simulink model "third_order"  (R2021b)
settings: Solver=VariableStepAuto  StartTime=0.0  StopTime=20  RelTol=1e-3
undefined symbols (not defined in the file): Amax, Amin, Ts, U, Vmax, Vmin
settings Model: Creator=11035  LastModifiedBy=11035

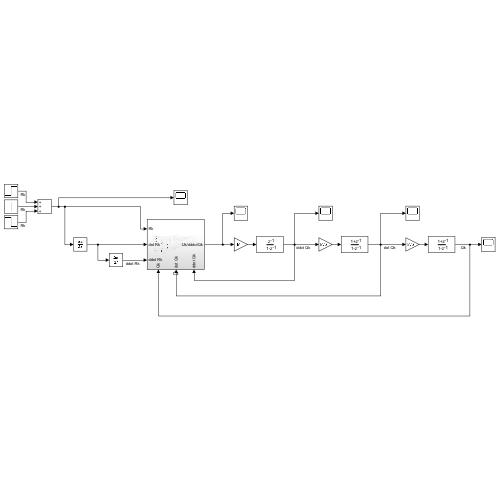
[thumbnail: Simulink's stored preview of the top-level diagram]
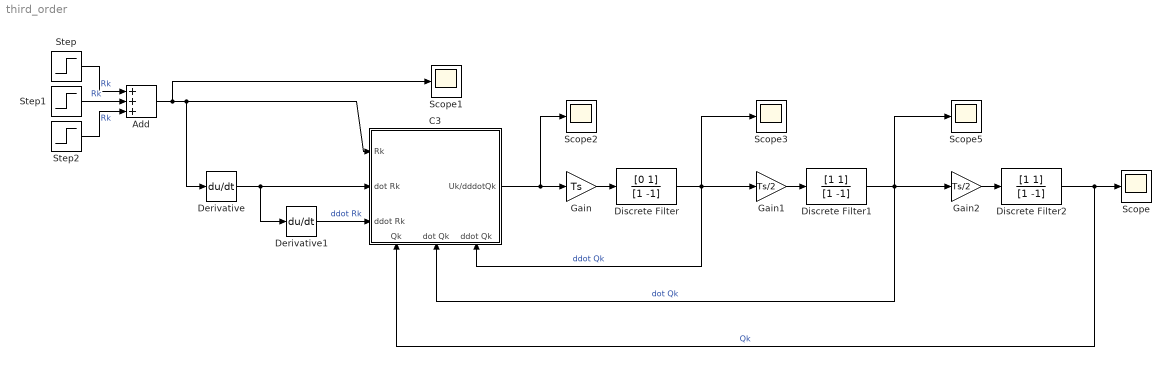
== system third_order ==
  Add : Sum  Inputs=+++
  C3 : Subsystem
      settings: PortSchema="{\"entries\":[{\"content\":{\"sides\":[{\"content\":{\"connectorIds\":[\"In1\",\"In2\",\"In3\"]},\"type\":\"ConnectorPlacement.EquallySpacedRectSide\",\"uuid\":\"716dbc1c-49b2-4cb8-9978-582acac14571\"},{\"content\":{\"connectorIds\":[\"Out1\"],\"side\":\"RIGHT\"},\"type\":\"ConnectorPlacement.EquallySpacedRectSide\",\"uuid\":\"02ab29e9-5fcc-4cd5-9c74-177b5082cb9c\"},{\"content\":{\"connectorIds\":[],\"side\":\"TOP\"},\"type\":\"ConnectorPlacement.EquallySpacedRectSide\",\"uuid\":\"01e65ab7-ae67-4bc4-815c-31b93fbda65a\"},{\"content\":{\"connectorIds\":[\"In4\",\"In5\",\"In6\"],\"side\":\"BOTTOM\"},\"type\":\"ConnectorPlacement.EquallySpacedRectSide\",\"uuid\":\"7a24d1a6-7a93-4ed1-ab59-9b35f53416c1\"}]},\"type\":\"ConnectorPlacement.EquallySpacedConnector\",\"uuid\":\"504bdbd8-79dc-4418-b775-c54dc6ccf1a1\"}],\"packageUris\":[\"http://schema.mathworks.com/mf0/Connector/R2020b\"],\"version\":\"1.0\"}"
  Derivative : Derivative
  Derivative1 : Derivative
  Discrete Filter : DiscreteFilter  Numerator=[0 1]  Denominator=[1 -1]
  Discrete Filter1 : DiscreteFilter  Numerator=[1 1]  Denominator=[1 -1]
  Discrete Filter2 : DiscreteFilter  Numerator=[1 1]  Denominator=[1 -1]
  Gain : Gain  Gain=Ts
  Gain1 : Gain  Gain=Ts/2
  Gain2 : Gain  Gain=Ts/2
  Scope{,1..3,5} (5 alike) : Scope
  Step : Step  After=4  SampleTime=0.001
  Step1 : Step  Time=7  After=6  SampleTime=0.001
  Step2 : Step  Time=13  After=-12  SampleTime=0.001
  wires:
  Gain1/1 -> Discrete Filter1/1
  Gain/1 -> Discrete Filter/1
  Discrete Filter1/1 -> C3/5(dot Qk), Gain2/1, Scope5/1  "dot Qk"
  Discrete Filter/1 -> C3/6(ddot Qk), Scope3/1, Gain1/1  "ddot Qk"
  Gain2/1 -> Discrete Filter2/1
  Discrete Filter2/1 -> Scope/1, C3/4(Qk)  "Qk"
  C3/1(Uk/dddotQk) -> Scope2/1, Gain/1
  Step1/1 -> Add/2  "Rk"
  Step/1 -> Add/1  "Rk"
  Step2/1 -> Add/3  "Rk"
  Add/1 -> Scope1/1, Derivative/1, C3/1(Rk)
  Derivative/1 -> C3/2(dot Rk), Derivative1/1
  Derivative1/1 -> C3/3(ddot Rk)  "ddot Rk"

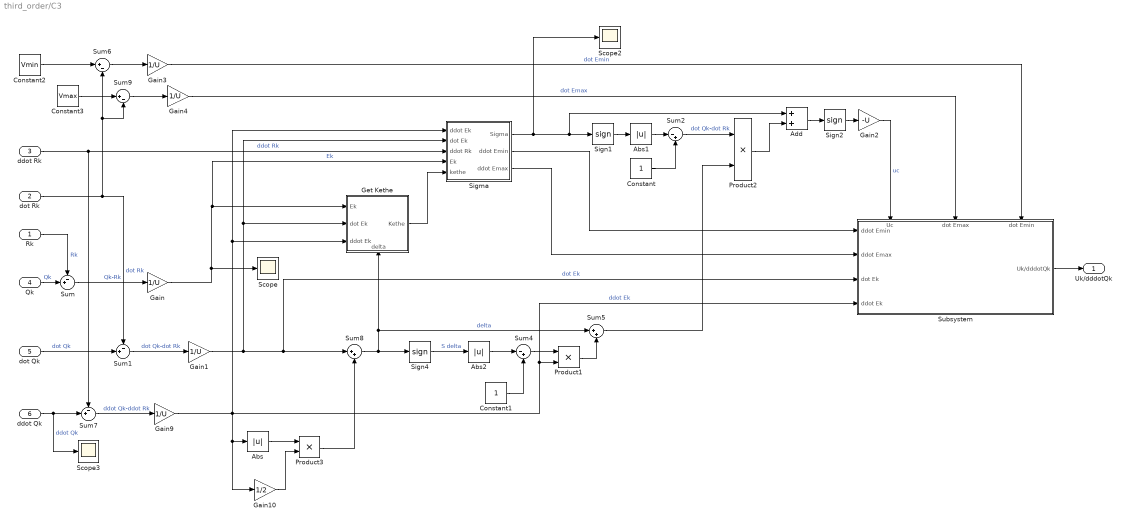
== system third_order/C3 ==
  Rk : Inport
  dot Rk : Inport  Port=2
  ddot Rk : Inport  Port=3
  Qk : Inport  Port=4
  dot Qk : Inport  Port=5
  ddot Qk : Inport  Port=6
  Abs : Abs
  Abs1 : Abs
  Abs2 : Abs
  Add : Sum
  Constant : Constant
  Constant1 : Constant
  Constant2 : Constant  Value=Vmin
  Constant3 : Constant  Value=Vmax
  Gain{,1,3..4,9} (5 alike) : Gain  Gain=1/U
  Gain10 : Gain  Gain=1/2
  Gain2 : Gain  Gain=-U
  Get Kethe : Subsystem
      settings: PortSchema="{\"entries\":[{\"content\":{\"sides\":[{\"content\":{\"connectorIds\":[\"In1\",\"In2\",\"In3\"]},\"type\":\"ConnectorPlacement.EquallySpacedRectSide\",\"uuid\":\"9252580f-5e9d-4265-be0b-e6bb3d304b20\"},{\"content\":{\"connectorIds\":[\"Out1\"],\"side\":\"RIGHT\"},\"type\":\"ConnectorPlacement.EquallySpacedRectSide\",\"uuid\":\"31fc0c8b-d7d5-4d3b-a162-fba5885efc54\"},{\"content\":{\"connectorIds\":[],\"side\":\"TOP\"},\"type\":\"ConnectorPlacement.EquallySpacedRectSide\",\"uuid\":\"1870fd8d-4272-45e5-86fe-422e41d939fb\"},{\"content\":{\"connectorIds\":[\"In4\"],\"side\":\"BOTTOM\"},\"type\":\"ConnectorPlacement.EquallySpacedRectSide\",\"uuid\":\"f1cc4331-f119-4651-8dc3-66dcf886f7f7\"}]},\"type\":\"ConnectorPlacement.EquallySpacedConnector\",\"uuid\":\"c093638c-209e-48b2-8550-858719cb62f2\"}],\"packageUris\":[\"http://schema.mathworks.com/mf0/Connector/R2020b\"],\"version\":\"1.0\"}"
  Product1 : Product
  Product2 : Product
  Product3 : Product
  Scope : Scope
  Scope2 : Scope
  Scope3 : Scope
  Sigma : Subsystem
  Sign1 : Signum
  Sign2 : Signum
  Sign4 : Signum
  Subsystem : Subsystem
      settings: PortSchema="{\"entries\":[{\"content\":{\"sides\":[{\"content\":{\"connectorIds\":[\"In1\",\"In2\",\"In3\",\"In4\"]},\"type\":\"ConnectorPlacement.EquallySpacedRectSide\",\"uuid\":\"36f01cd8-9b20-4b96-874e-21a8302aaf05\"},{\"content\":{\"connectorIds\":[\"Out1\"],\"side\":\"RIGHT\"},\"type\":\"ConnectorPlacement.EquallySpacedRectSide\",\"uuid\":\"aff3e783-8ccd-4767-9c32-464e65717a87\"},{\"content\":{\"connectorIds\":[\"In5\",\"In6\",\"In7\"],\"side\":\"TOP\"},\"type\":\"ConnectorPlacement.EquallySpacedRectSide\",\"uuid\":\"c94c5949-abb6-4ff8-bb3f-d90959b8a55f\"}]},\"type\":\"ConnectorPlacement.EquallySpacedConnector\",\"uuid\":\"91cab301-bc0d-448e-a06d-cf998fceab8f\"}],\"packageUris\":[\"http://schema.mathworks.com/mf0/Connector/R2020b\"],\"version\":\"1.0\"}"
  Sum : Sum  Inputs=-+|
  Sum1 : Sum  Inputs=-+|
  Sum2 : Sum  Inputs=|-+
  Sum4 : Sum  Inputs=|-+
  Sum5 : Sum  Inputs=|++
  Sum6 : Sum  Inputs=|+-
  Sum7 : Sum  Inputs=-+|
  Sum8 : Sum  Inputs=|++
  Sum9 : Sum  Inputs=|+-
  Uk/dddotQk : Outport
  wires:
  Rk/1 -> Sum/1  "Rk"
  Qk/1 -> Sum/2  "Qk"
  Sum/1 -> Gain/1  "Qk-Rk"
  dot Qk/1 -> Sum1/2  "dot Qk"
  Sum1/1 -> Gain1/1  "dot Qk-dot Rk"
  dot Rk/1 -> Sum9/2, Sum6/2, Sum1/1  "dot Rk"
  ddot Qk/1 -> Scope3/1, Sum7/2  "ddot Qk"
  Sum7/1 -> Gain9/1  "ddot Qk-ddot Rk"
  Abs/1 -> Product3/1
  Gain10/1 -> Product3/2
  Product3/1 -> Sum8/2
  Sum8/1 -> Sign4/1, Sum5/1, Get Kethe/4(delta)  "delta"
  Sign4/1 -> Abs2/1  "S delta"
  Gain1/1 -> Sigma/2(dot Ek), Get Kethe/2(dot Ek), Sum8/1, Subsystem/3(dot Ek)  "dot Ek"
  Gain9/1 -> Gain10/1, Abs/1, Product1/2, Subsystem/4(ddot Ek), Get Kethe/3(ddot Ek), Sigma/1(ddot Ek)  "ddot Ek"
  ddot Rk/1 -> Sum7/1, Sigma/3(ddot Rk)  "ddot Rk"
  Gain/1 -> Scope/1, Sigma/4(Ek), Get Kethe/1(Ek)  "Ek"
  Sigma/1(Sigma) -> Scope2/1, Add/1, Sign1/1
  Sign1/1 -> Abs1/1
  Abs1/1 -> Sum2/1
  Constant/1 -> Sum2/2
  Constant1/1 -> Sum4/2
  Abs2/1 -> Sum4/1
  Sum4/1 -> Product1/1
  Product1/1 -> Sum5/2
  Sigma/2(ddot Emin) -> Subsystem/1(ddot Emin)
  Sigma/3(ddot Emax) -> Subsystem/2(ddot Emax)
  Subsystem/1(Uk/dddotQk) -> Uk/dddotQk/1
  Constant2/1 -> Sum6/1
  Sum6/1 -> Gain3/1
  Gain3/1 -> Subsystem/7(dot Emin)  "dot Emin"
  Constant3/1 -> Sum9/1
  Sum9/1 -> Gain4/1
  Gain4/1 -> Subsystem/6(dot Emax)  "dot Emax"
  Sum2/1 -> Product2/1  "dot Qk-dot Rk"
  Sum5/1 -> Product2/2
  Product2/1 -> Add/2
  Add/1 -> Sign2/1
  Gain2/1 -> Subsystem/5("Uc ")  "uc"
  Get Kethe/1(Kethe) -> Sigma/5(kethe)
  Sign2/1 -> Gain2/1

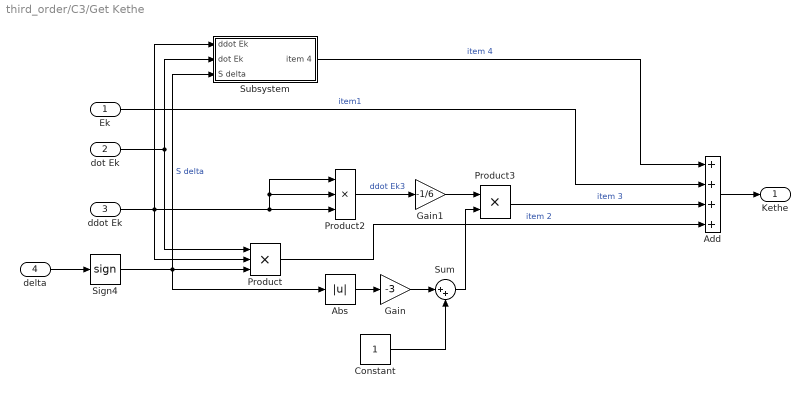
== system third_order/C3/Get Kethe ==
  Ek : Inport
  dot Ek : Inport  Port=2
  ddot Ek : Inport  Port=3
  delta : Inport  Port=4
  Abs : Abs
  Add : Sum  Inputs=++++
  Constant : Constant
  Gain : Gain  Gain=-3
  Gain1 : Gain  Gain=-1/6
  Product : Product  Inputs=3
  Product2 : Product  Inputs=3
  Product3 : Product
  Sign4 : Signum
  Subsystem : Subsystem
  Sum : Sum  Inputs=|++
  Kethe : Outport
  wires:
  delta/1 -> Sign4/1
  dot Ek/1 -> Subsystem/2(dot Ek), Product/1
  ddot Ek/1 -> Product2/2, Product2/1, Product2/3, Subsystem/1(ddot Ek), Product/2
  Product2/1 -> Gain1/1  "ddot Ek3"
  Product/1 -> Add/4  "item 2"
  Sign4/1 -> Subsystem/3(S delta), Product/3, Abs/1  "S delta"
  Abs/1 -> Gain/1
  Gain/1 -> Sum/1
  Constant/1 -> Sum/2
  Gain1/1 -> Product3/1
  Sum/1 -> Product3/2
  Product3/1 -> Add/3  "item 3"
  Subsystem/1(item 4) -> Add/1  "item 4"
  Ek/1 -> Add/2  "item1"
  Add/1 -> Kethe/1

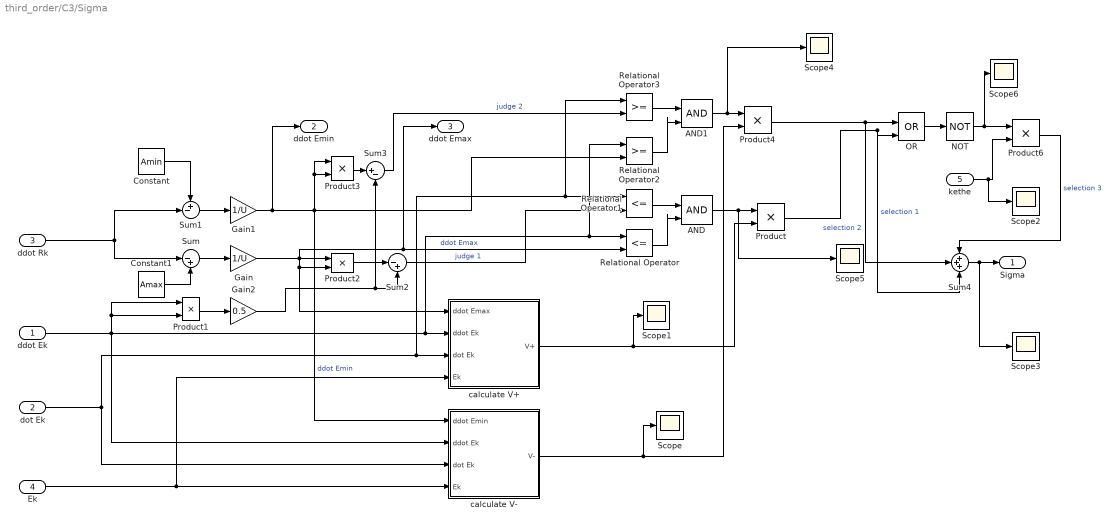
== system third_order/C3/Sigma ==
  ddot Ek : Inport
  dot Ek : Inport  Port=2
  ddot Rk : Inport  Port=3
  Ek : Inport  Port=4
  kethe : Inport  Port=5
  AND : Logic  IconShape=distinctive  AllPortsSameDT=off  OutDataTypeStr=boolean
  AND1 : Logic  IconShape=distinctive  AllPortsSameDT=off  OutDataTypeStr=boolean
  Constant : Constant  Value=Amin
  Constant1 : Constant  Value=Amax
  Gain : Gain  Gain=1/U
  Gain1 : Gain  Gain=1/U
  Gain2 : Gain  Gain=0.5
  NOT : Logic  Operator=NOT  IconShape=distinctive  AllPortsSameDT=off  OutDataTypeStr=boolean
  OR : Logic  Operator=OR  IconShape=distinctive  AllPortsSameDT=off  OutDataTypeStr=boolean
  Product{,1..4,6} (6 alike) : Product
  Relational Operator : RelationalOperator  Operator=<=  OutDataTypeStr=boolean  RndMeth=Simplest
  Relational Operator1 : RelationalOperator  Operator=<=  OutDataTypeStr=boolean  RndMeth=Simplest
  Relational Operator2 : RelationalOperator  OutDataTypeStr=boolean  RndMeth=Simplest
  Relational Operator3 : RelationalOperator  OutDataTypeStr=boolean  RndMeth=Simplest
  Scope{,1..6} (7 alike) : Scope
  Sum : Sum  Inputs=|-+
  Sum1 : Sum  Inputs=+-|
  Sum2 : Sum  Inputs=|-+
  Sum3 : Sum  Inputs=|+-
  Sum4 : Sum  Inputs=+++
  calculate V+ : Subsystem
  calculate V- : Subsystem
  Sigma : Outport
  ddot Emin : Outport  Port=2
  ddot Emax : Outport  Port=3
  wires:
  Sum1/1 -> Gain1/1
  Constant/1 -> Sum1/1
  Sum/1 -> Gain/1
  ddot Rk/1 -> Sum/1, Sum1/2
  Constant1/1 -> Sum/2
  dot Ek/1 -> calculate V-/3(dot Ek), Relational Operator3/1, Relational Operator1/1, calculate V+/3(dot Ek)
  Ek/1 -> calculate V-/4(Ek), calculate V+/4(Ek)
  Gain1/1 -> Relational Operator2/2, Product3/2, Product3/1, calculate V-/1(ddot Emin), ddot Emin/1  "ddot Emin"
  Gain/1 -> Product2/1, calculate V+/1(ddot Emax), Product2/2, ddot Emax/1, Relational Operator/2  "ddot Emax"
  Product1/1 -> Gain2/1
  Product2/1 -> Sum2/1
  Gain2/1 -> Sum3/2, Sum2/2
  calculate V+/1(V+) -> Scope1/1, Product/2
  Sum2/1 -> Relational Operator1/2  "judge 1"
  Product3/1 -> Sum3/1
  Sum3/1 -> Relational Operator3/2  "judge 2"
  calculate V-/1(V-) -> Scope/1, Product4/2
  ddot Ek/1 -> Product1/1, Product1/2, Relational Operator2/1, Relational Operator/1, calculate V+/2(ddot Ek), calculate V-/2(ddot Ek)
  Relational Operator1/1 -> AND/1
  Relational Operator/1 -> AND/2
  AND/1 -> Scope5/1, Product/1
  Product/1 -> Sum4/3, OR/2  "selection 1"
  Relational Operator3/1 -> AND1/1
  Relational Operator2/1 -> AND1/2
  AND1/1 -> Scope4/1, Product4/1
  OR/1 -> NOT/1
  NOT/1 -> Scope6/1, Product6/1
  kethe/1 -> Scope2/1, Product6/2
  Product6/1 -> Sum4/1  "selection 3"
  Product4/1 -> Sum4/2, OR/1  "selection 2"
  Sum4/1 -> Scope3/1, Sigma/1

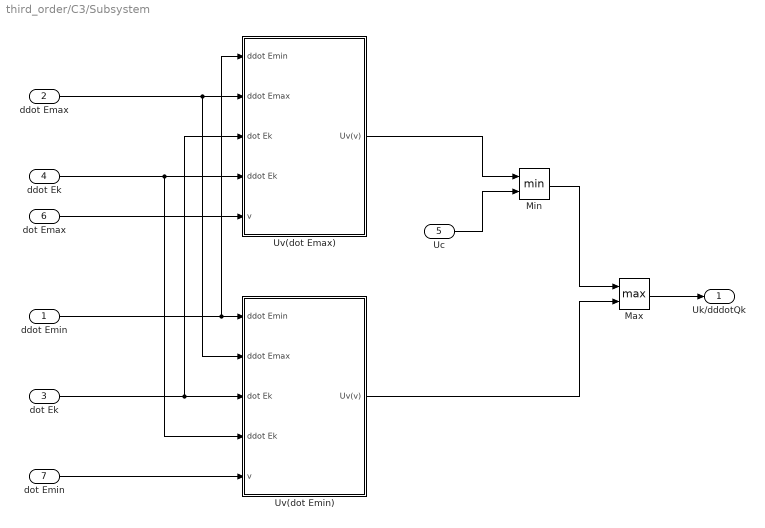
== system third_order/C3/Subsystem ==
  ddot Emin : Inport
  ddot Emax : Inport  Port=2
  dot Ek : Inport  Port=3
  ddot Ek : Inport  Port=4
  "Uc " : Inport  Port=5
  dot Emax : Inport  Port=6
  dot Emin : Inport  Port=7
  Max : MinMax  Function=max  Inputs=2
  Min : MinMax  Inputs=2
  Uv(dot Emax) : Subsystem
  Uv(dot Emin) : Subsystem
  Uk/dddotQk : Outport
  wires:
  ddot Emin/1 -> Uv(dot Emax)/1(ddot Emin), Uv(dot Emin)/1(ddot Emin)
  ddot Emax/1 -> Uv(dot Emin)/2(ddot Emax), Uv(dot Emax)/2(ddot Emax)
  dot Ek/1 -> Uv(dot Emin)/3(dot Ek), Uv(dot Emax)/3(dot Ek)
  ddot Ek/1 -> Uv(dot Emin)/4(ddot Ek), Uv(dot Emax)/4(ddot Ek)
  "Uc "/1 -> Min/2
  Uv(dot Emax)/1(Uv(v)) -> Min/1
  Min/1 -> Max/1
  Uv(dot Emin)/1(Uv(v)) -> Max/2
  Max/1 -> Uk/dddotQk/1
  dot Emax/1 -> Uv(dot Emax)/5("v ")
  dot Emin/1 -> Uv(dot Emin)/5("v ")

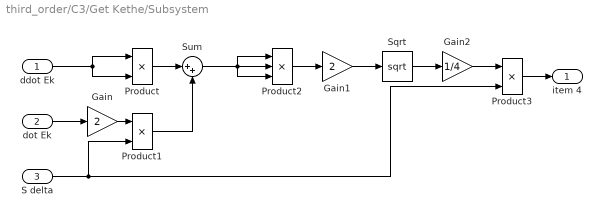
== system third_order/C3/Get Kethe/Subsystem ==
  ddot Ek : Inport
  dot Ek : Inport  Port=2
  S delta : Inport  Port=3
  Gain : Gain  Gain=2
  Gain1 : Gain  Gain=2
  Gain2 : Gain  Gain=1/4
  Product : Product
  Product1 : Product
  Product2 : Product  Inputs=3
  Product3 : Product
  Sqrt : Sqrt  SaturateOnIntegerOverflow=on
  Sum : Sum  Inputs=|++
  item 4 : Outport
  wires:
  ddot Ek/1 -> Product/1, Product/2
  dot Ek/1 -> Gain/1
  Gain/1 -> Product1/1
  S delta/1 -> Product3/2, Product1/2
  Product/1 -> Sum/1
  Product1/1 -> Sum/2
  Sum/1 -> Product2/3, Product2/1, Product2/2
  Product2/1 -> Gain1/1
  Gain1/1 -> Sqrt/1
  Sqrt/1 -> Gain2/1
  Gain2/1 -> Product3/1
  Product3/1 -> item 4/1

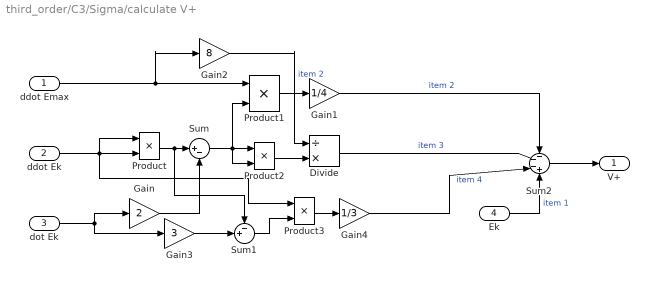
== system third_order/C3/Sigma/calculate V+ ==
  ddot Emax : Inport
  ddot Ek : Inport  Port=2
  dot Ek : Inport  Port=3
  Ek : Inport  Port=4
  Divide : Product  Inputs=/*
  Gain : Gain  Gain=2
  Gain1 : Gain  Gain=1/4
  Gain2 : Gain  Gain=8
  Gain3 : Gain  Gain=3
  Gain4 : Gain  Gain=1/3
  Product{,1..3} (4 alike) : Product
  Sum : Sum  Inputs=|+-
  Sum1 : Sum  Inputs=-+|
  Sum2 : Sum  Inputs=---+
  V+ : Outport
  wires:
  Ek/1 -> Sum2/4  "item 1"
  ddot Ek/1 -> Product3/1, Product/2, Product/1
  Product/1 -> Sum1/1, Sum/1
  Gain/1 -> Sum/2
  ddot Emax/1 -> Gain2/1, Product1/1
  Product1/1 -> Gain1/1
  Gain1/1 -> Sum2/1  "item 2"
  Sum/1 -> Product1/2, Product2/2, Product2/1
  Product2/1 -> Divide/2
  Gain2/1 -> Divide/1  "item 2"
  Divide/1 -> Sum2/2  "item 3"
  dot Ek/1 -> Gain/1, Gain3/1
  Gain3/1 -> Sum1/2
  Sum1/1 -> Product3/2
  Product3/1 -> Gain4/1
  Gain4/1 -> Sum2/3  "item 4"
  Sum2/1 -> V+/1

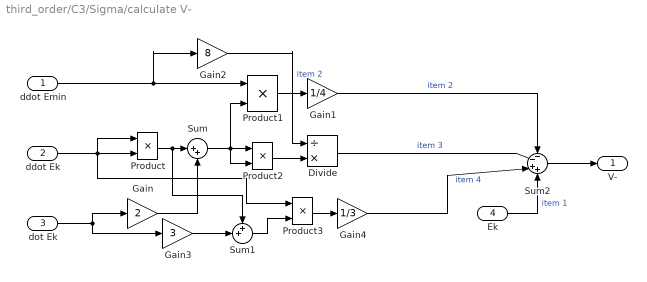
== system third_order/C3/Sigma/calculate V- ==
  ddot Emin : Inport
  ddot Ek : Inport  Port=2
  dot Ek : Inport  Port=3
  Ek : Inport  Port=4
  Divide : Product  Inputs=/*
  Gain : Gain  Gain=2
  Gain1 : Gain  Gain=1/4
  Gain2 : Gain  Gain=8
  Gain3 : Gain  Gain=3
  Gain4 : Gain  Gain=1/3
  Product{,1..3} (4 alike) : Product
  Sum : Sum  Inputs=|++
  Sum1 : Sum  Inputs=++|
  Sum2 : Sum  Inputs=--++
  V- : Outport
  wires:
  Ek/1 -> Sum2/4  "item 1"
  Product/1 -> Sum1/1, Sum/1
  Gain/1 -> Sum/2
  ddot Emin/1 -> Gain2/1, Product1/1
  Product1/1 -> Gain1/1
  Gain1/1 -> Sum2/1  "item 2"
  Sum/1 -> Product1/2, Product2/1, Product2/2
  Product2/1 -> Divide/2
  Gain2/1 -> Divide/1  "item 2"
  Divide/1 -> Sum2/2  "item 3"
  Gain3/1 -> Sum1/2
  Sum1/1 -> Product3/2
  Product3/1 -> Gain4/1
  Gain4/1 -> Sum2/3  "item 4"
  Sum2/1 -> V-/1
  ddot Ek/1 -> Product3/1, Product/2, Product/1
  dot Ek/1 -> Gain3/1, Gain/1

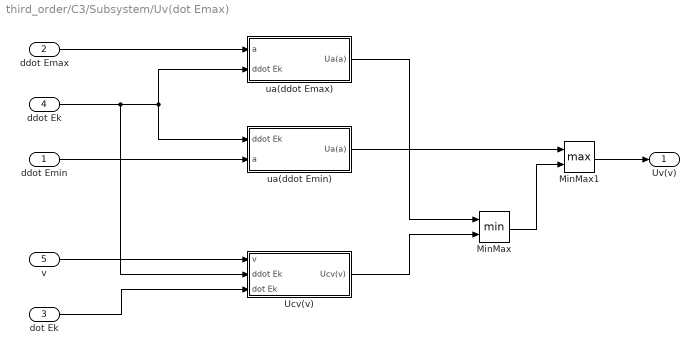
== system third_order/C3/Subsystem/Uv(dot Emax) ==
  ddot Emin : Inport
  ddot Emax : Inport  Port=2
  dot Ek : Inport  Port=3
  ddot Ek : Inport  Port=4
  "v " : Inport  Port=5
  MinMax : MinMax  Inputs=2
  MinMax1 : MinMax  Function=max  Inputs=2
  Ucv(v) : Subsystem
  ua(ddot Emax) : Subsystem
  ua(ddot Emin) : Subsystem
  Uv(v) : Outport
  wires:
  ddot Ek/1 -> Ucv(v)/2(ddot Ek), ua(ddot Emin)/1(ddot Ek), ua(ddot Emax)/2(ddot Ek)
  ddot Emax/1 -> ua(ddot Emax)/1(a)
  ddot Emin/1 -> ua(ddot Emin)/2(a)
  "v "/1 -> Ucv(v)/1(v)
  dot Ek/1 -> Ucv(v)/3(dot Ek)
  Ucv(v)/1(Ucv(v)) -> MinMax/2
  ua(ddot Emax)/1(Ua(a)) -> MinMax/1
  ua(ddot Emin)/1(Ua(a)) -> MinMax1/1
  MinMax/1 -> MinMax1/2
  MinMax1/1 -> Uv(v)/1

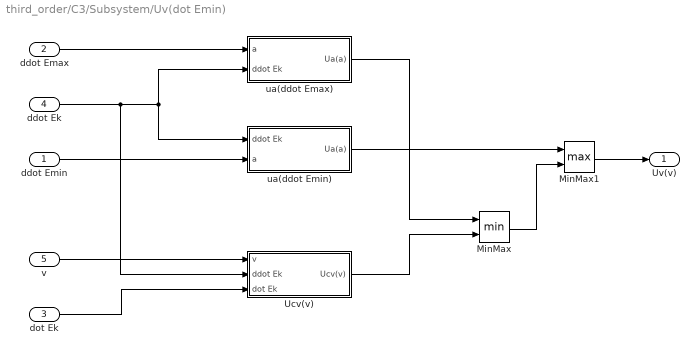
== system third_order/C3/Subsystem/Uv(dot Emin) ==
  ddot Emin : Inport
  ddot Emax : Inport  Port=2
  dot Ek : Inport  Port=3
  ddot Ek : Inport  Port=4
  "v " : Inport  Port=5
  MinMax : MinMax  Inputs=2
  MinMax1 : MinMax  Function=max  Inputs=2
  Ucv(v) : Subsystem
  ua(ddot Emax) : Subsystem
  ua(ddot Emin) : Subsystem
  Uv(v) : Outport
  wires:
  ddot Ek/1 -> Ucv(v)/2(ddot Ek), ua(ddot Emin)/1(ddot Ek), ua(ddot Emax)/2(ddot Ek)
  ddot Emax/1 -> ua(ddot Emax)/1(a)
  ddot Emin/1 -> ua(ddot Emin)/2(a)
  "v "/1 -> Ucv(v)/1(v)
  dot Ek/1 -> Ucv(v)/3(dot Ek)
  Ucv(v)/1(Ucv(v)) -> MinMax/2
  ua(ddot Emax)/1(Ua(a)) -> MinMax/1
  ua(ddot Emin)/1(Ua(a)) -> MinMax1/1
  MinMax/1 -> MinMax1/2
  MinMax1/1 -> Uv(v)/1

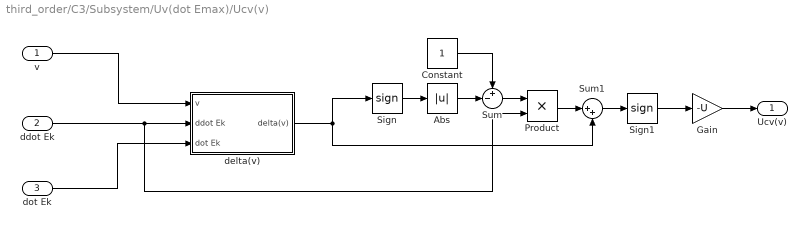
== system third_order/C3/Subsystem/Uv(dot Emax)/Ucv(v) ==
  v : Inport
  ddot Ek : Inport  Port=2
  dot Ek : Inport  Port=3
  Abs : Abs
  Constant : Constant
  Gain : Gain  Gain=-U
  Product : Product
  Sign : Signum
  Sign1 : Signum
  Sum : Sum  Inputs=+-|
  Sum1 : Sum  Inputs=|++
  delta(v) : Subsystem
  Ucv(v) : Outport
  wires:
  ddot Ek/1 -> Product/2, delta(v)/2(ddot Ek)
  dot Ek/1 -> delta(v)/3(dot Ek)
  v/1 -> delta(v)/1(v)
  Sign/1 -> Abs/1
  Abs/1 -> Sum/2
  Constant/1 -> Sum/1
  Sum/1 -> Product/1
  Product/1 -> Sum1/1
  delta(v)/1(delta(v)) -> Sum1/2, Sign/1
  Sum1/1 -> Sign1/1
  Sign1/1 -> Gain/1
  Gain/1 -> Ucv(v)/1

== system third_order/C3/Subsystem/Uv(dot Emax)/ua(ddot Emax) ==
  a : Inport
  ddot Ek : Inport  Port=2
  Gain : Gain  Gain=-U
  Sign : Signum
  Sum : Sum  Inputs=+-|
  Ua(a) : Outport
  wires:
  a/1 -> Sum/2
  ddot Ek/1 -> Sum/1
  Sum/1 -> Sign/1
  Sign/1 -> Gain/1
  Gain/1 -> Ua(a)/1

== system third_order/C3/Subsystem/Uv(dot Emax)/ua(ddot Emin) ==
  ddot Ek : Inport
  a : Inport  Port=2
  Gain : Gain  Gain=-U
  Sign : Signum
  Sum : Sum  Inputs=+-|
  Ua(a) : Outport
  wires:
  a/1 -> Sum/2
  ddot Ek/1 -> Sum/1
  Sum/1 -> Sign/1
  Sign/1 -> Gain/1
  Gain/1 -> Ua(a)/1

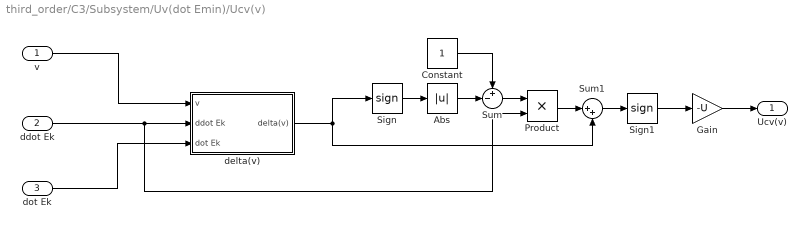
== system third_order/C3/Subsystem/Uv(dot Emin)/Ucv(v) ==
  v : Inport
  ddot Ek : Inport  Port=2
  dot Ek : Inport  Port=3
  Abs : Abs
  Constant : Constant
  Gain : Gain  Gain=-U
  Product : Product
  Sign : Signum
  Sign1 : Signum
  Sum : Sum  Inputs=+-|
  Sum1 : Sum  Inputs=|++
  delta(v) : Subsystem
  Ucv(v) : Outport
  wires:
  ddot Ek/1 -> Product/2, delta(v)/2(ddot Ek)
  dot Ek/1 -> delta(v)/3(dot Ek)
  v/1 -> delta(v)/1(v)
  Sign/1 -> Abs/1
  Abs/1 -> Sum/2
  Constant/1 -> Sum/1
  Sum/1 -> Product/1
  Product/1 -> Sum1/1
  delta(v)/1(delta(v)) -> Sum1/2, Sign/1
  Sum1/1 -> Sign1/1
  Sign1/1 -> Gain/1
  Gain/1 -> Ucv(v)/1

== system third_order/C3/Subsystem/Uv(dot Emin)/ua(ddot Emax) ==
  a : Inport
  ddot Ek : Inport  Port=2
  Gain : Gain  Gain=-U
  Sign : Signum
  Sum : Sum  Inputs=+-|
  Ua(a) : Outport
  wires:
  a/1 -> Sum/2
  ddot Ek/1 -> Sum/1
  Sum/1 -> Sign/1
  Sign/1 -> Gain/1
  Gain/1 -> Ua(a)/1

== system third_order/C3/Subsystem/Uv(dot Emin)/ua(ddot Emin) ==
  ddot Ek : Inport
  a : Inport  Port=2
  Gain : Gain  Gain=-U
  Sign : Signum
  Sum : Sum  Inputs=+-|
  Ua(a) : Outport
  wires:
  a/1 -> Sum/2
  ddot Ek/1 -> Sum/1
  Sum/1 -> Sign/1
  Sign/1 -> Gain/1
  Gain/1 -> Ua(a)/1

== system third_order/C3/Subsystem/Uv(dot Emax)/Ucv(v)/delta(v) ==
  v : Inport
  ddot Ek : Inport  Port=2
  dot Ek : Inport  Port=3
  Abs : Abs
  Gain : Gain  Gain=2
  Product : Product
  Sum : Sum  Inputs=-+|
  Sum1 : Sum  Inputs=++|
  delta(v) : Outport
  wires:
  v/1 -> Sum/1
  dot Ek/1 -> Sum/2
  Sum/1 -> Gain/1
  ddot Ek/1 -> Abs/1, Product/1
  Abs/1 -> Product/2
  Product/1 -> Sum1/2
  Gain/1 -> Sum1/1
  Sum1/1 -> delta(v)/1

== system third_order/C3/Subsystem/Uv(dot Emin)/Ucv(v)/delta(v) ==
  v : Inport
  ddot Ek : Inport  Port=2
  dot Ek : Inport  Port=3
  Abs : Abs
  Gain : Gain  Gain=2
  Product : Product
  Sum : Sum  Inputs=-+|
  Sum1 : Sum  Inputs=++|
  delta(v) : Outport
  wires:
  v/1 -> Sum/1
  dot Ek/1 -> Sum/2
  Sum/1 -> Gain/1
  Abs/1 -> Product/2
  Product/1 -> Sum1/2
  Gain/1 -> Sum1/1
  Sum1/1 -> delta(v)/1
  ddot Ek/1 -> Abs/1, Product/1
